simulink subsystem "Dist_Models_Integrator_2"  (R2025b)
settings: Solver=VariableStepAuto  StartTime=0.0  StopTime=10.0  RelTol=1e-3
undefined symbols (not defined in the file or in its folder): DiscIntNeverNeededParam, x0
settings Model: Creator=pplat  LastModifiedBy=pplat

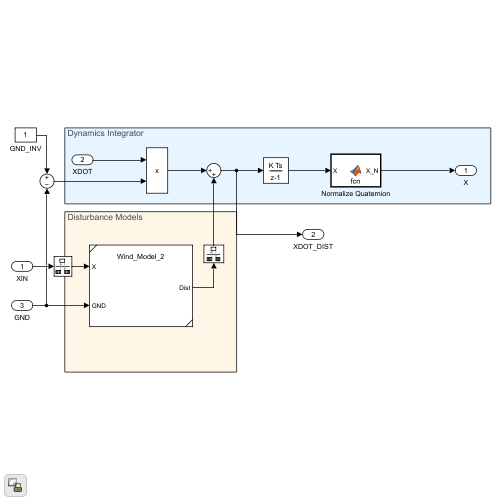
[thumbnail: Simulink's stored preview of the top-level diagram]
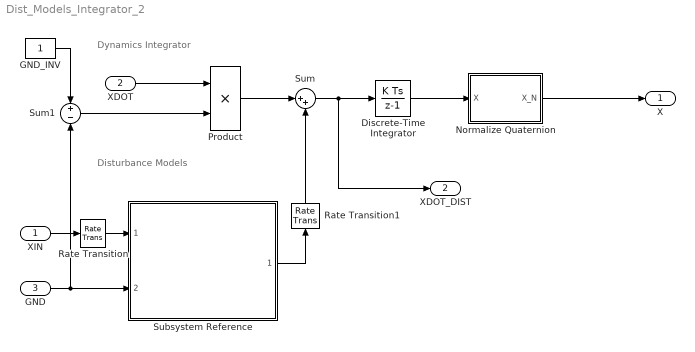
== system Dist_Models_Integrator_2 ==
  note: Dynamics Integrator
  note: Disturbance Models
  XIN : Inport
  XDOT : Inport  Port=2  PortDimensions=[15,1]
  GND : Inport  Port=3
  Discrete-Time Integrator : DiscreteIntegrator  InitialCondition=x0  SampleTime=-1  ICPrevOutput=DiscIntNeverNeededParam  ICPrevScaledInput=DiscIntNeverNeededParam
  GND_INV : Constant
  Normalize Quaternion : MATLAB Function  TreatAsAtomicUnit=on
  Product : Product
  Rate Transition : RateTransition  InitialCondition=[1; zeros(14,1)]  OutPortSampleTime=1/50
  Rate Transition1 : RateTransition  InitialCondition=[zeros(15,1)]  OutPortSampleTime=dt_SIM
  Subsystem Reference : Subsystem  ReferencedSubsystem=Wind_Model_2
  Sum : Sum  Inputs=|++
  Sum1 : Sum  Inputs=+|-
  X : Outport
  XDOT_DIST : Outport  Port=2
  wires:
  Sum/1 -> Discrete-Time Integrator/1, XDOT_DIST/1
  Subsystem Reference/1 -> Rate Transition1/1
  XDOT/1 -> Product/1
  Discrete-Time Integrator/1 -> Normalize Quaternion/1(X)
  XIN/1 -> Rate Transition/1
  GND/1 -> Subsystem Reference/2, Sum1/2
  GND_INV/1 -> Sum1/1
  Product/1 -> Sum/1
  Normalize Quaternion/1(X_N) -> X/1
  Sum1/1 -> Product/2
  Rate Transition/1 -> Subsystem Reference/1
  Rate Transition1/1 -> Sum/2

== matlab function Dist_Models_Integrator_2/Normalize Quaternion ==
  data: X input; X_N output
function X_N = fcn(X)
X_N = [X(1:4) / norm(X(1:4)); X(5:end)];
